simulink model "FxLMS_Sys"  (R2024b)
settings: Solver=FixedStepDiscrete  StartTime=0.0  StopTime=10  FixedStep=1/48000  RelTol=1e-3
values from neighbouring files (symbols this model uses):
  sim_p = conv(sim_s,sim_f)    [FxLMS_algo_sim.m]
  sim_s = [0.5 0.5 -0.3 -0.3 -0.2 -0.2]    [FxLMS_algo_sim.m]
undefined symbols (not defined in the file or in its folder): dspblkCoreblockFVToolHelper, gcbh
libraries: dspadpt3 x1, dspfdesign x1, dspsrcs4 x1
settings Model: PacingRate=10  Creator=shaar  LastModifiedBy=shaar

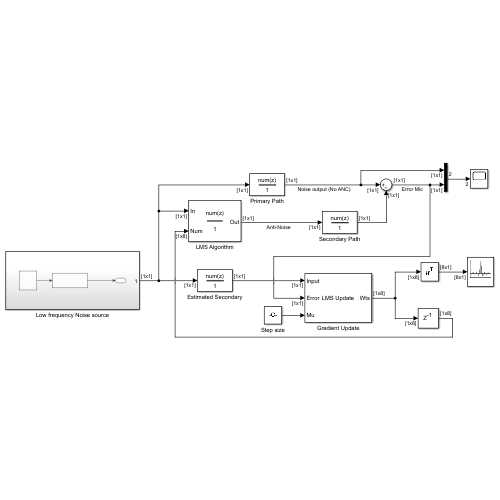
[thumbnail: Simulink's stored preview of the top-level diagram]
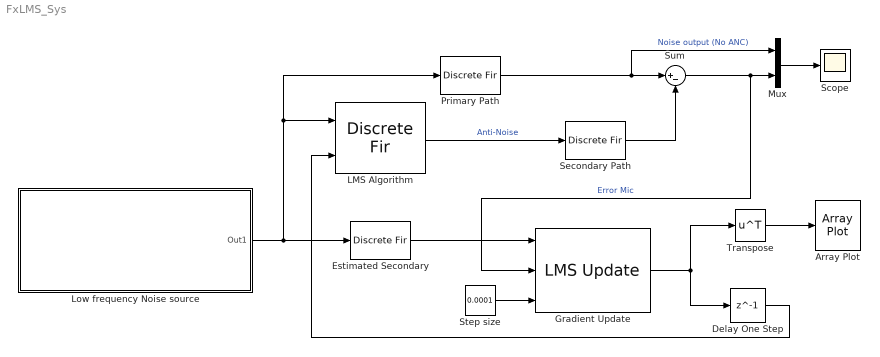
== system FxLMS_Sys ==
  Array Plot : ArrayPlot  WindowPosition=[49.000000,142.000000,800.000000,500.000000,]  ScopeFrameLocation=window  YLimits=[-0.0053 0.0054]
  Delay One Step : Delay  DelayLength=1
  Estimated Secondary : DiscreteFir  LoadFcn=dspblkCoreblockFVToolHelper(gcbh,'load');  Coefficients=sim_s
      settings: CopyFcn=dspblkCoreblockFVToolHelper(gcbh,'copy');  DeleteFcn=dspblkCoreblockFVToolHelper(gcbh,'close');  ModelCloseFcn=dspblkCoreblockFVToolHelper(gcbh,'close');  PreSaveFcn=dspblkCoreblockFVToolHelper(gcbh,'presave');  PostSaveFcn=dspblkCoreblockFVToolHelper(gcbh,'postsave');  CloseFcn=dspblkCoreblockFVToolHelper(gcbh,'close');
  Gradient Update : dspadpt3/LMS Update  Method=Normalized LMS  Length=8  NumFilters=1  StepSizeSource=Input port  StepSize=0.1  LeakageFactor=1.0  InitialConditions=0  AdaptiveFilterMode=Tapped delay-line FIR filter  EnableAdaptInput=off  EnableResetInput=off  SimulateUsing=Interpreted execution
  LMS Algorithm : DiscreteFir  LoadFcn=dspblkCoreblockFVToolHelper(gcbh,'load');  CoefSource=Input port
      settings: CopyFcn=dspblkCoreblockFVToolHelper(gcbh,'copy');  DeleteFcn=dspblkCoreblockFVToolHelper(gcbh,'close');  ModelCloseFcn=dspblkCoreblockFVToolHelper(gcbh,'close');  PreSaveFcn=dspblkCoreblockFVToolHelper(gcbh,'presave');  PostSaveFcn=dspblkCoreblockFVToolHelper(gcbh,'postsave');  CloseFcn=dspblkCoreblockFVToolHelper(gcbh,'close');  InputPortMap=u0,u1
  Low frequency Noise source : Subsystem
  Mux : Mux  Inputs=2
  Primary Path : DiscreteFir  LoadFcn=dspblkCoreblockFVToolHelper(gcbh,'load');  Coefficients=sim_p
      settings: CopyFcn=dspblkCoreblockFVToolHelper(gcbh,'copy');  DeleteFcn=dspblkCoreblockFVToolHelper(gcbh,'close');  ModelCloseFcn=dspblkCoreblockFVToolHelper(gcbh,'close');  PreSaveFcn=dspblkCoreblockFVToolHelper(gcbh,'presave');  PostSaveFcn=dspblkCoreblockFVToolHelper(gcbh,'postsave');  CloseFcn=dspblkCoreblockFVToolHelper(gcbh,'close');
  Scope : Scope
  Secondary Path : DiscreteFir  LoadFcn=dspblkCoreblockFVToolHelper(gcbh,'load');  Coefficients=sim_s
      settings: CopyFcn=dspblkCoreblockFVToolHelper(gcbh,'copy');  DeleteFcn=dspblkCoreblockFVToolHelper(gcbh,'close');  ModelCloseFcn=dspblkCoreblockFVToolHelper(gcbh,'close');  PreSaveFcn=dspblkCoreblockFVToolHelper(gcbh,'presave');  PostSaveFcn=dspblkCoreblockFVToolHelper(gcbh,'postsave');  CloseFcn=dspblkCoreblockFVToolHelper(gcbh,'close');
  Step size : Constant  Value=0.0001
  Sum : Sum  Inputs=|+-
  Transpose : Math  Operator=transpose
  wires:
  Primary Path/1 -> Mux/1, Sum/1  "Noise output (No ANC)"
  Secondary Path/1 -> Sum/2
  LMS Algorithm/1 -> Secondary Path/1  "Anti-Noise"
  Sum/1 -> Mux/2, Gradient Update/2  "Error Mic"
  Gradient Update/1 -> Delay One Step/1, Transpose/1
  Delay One Step/1 -> LMS Algorithm/2
  Transpose/1 -> Array Plot/1
  Step size/1 -> Gradient Update/3
  Estimated Secondary/1 -> Gradient Update/1
  Mux/1 -> Scope/1
  Low frequency Noise source/1(Out1) -> Estimated Secondary/1, LMS Algorithm/1, Primary Path/1

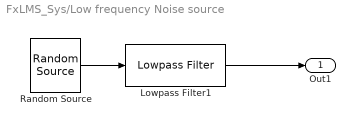
== system FxLMS_Sys/Low frequency Noise source ==
  Lowpass Filter1 : dspfdesign/Lowpass Filter  FilterType=FIR  DesignForMinimumOrder=on  FilterOrder=50  PassbandFrequency=0.0125  StopbandFrequency=0.0167  PassbandRipple=0.1  StopbandAttenuation=80  SampleRateMode=Use normalized frequency (0 to 1)  SampleRate=44100  SimulateUsing=Interpreted execution  roundingMode=Floor  coeffsDataTypeStr=fixdt(1,16)
  Random Source : dspsrcs4/Random Source  SrcType=Uniform  MinVal=-0.05  MaxVal=0.05  MeanVal=0  VarVal=1  RepMode=Specify seed  rawSeed=1  IsInherit=off  SampTime=1/48000  SampFrame=1  OutComplex=Real  DataType=double  SimulateUsing=Interpreted execution
  Out1 : Outport
  wires:
  Random Source/1 -> Lowpass Filter1/1
  Lowpass Filter1/1 -> Out1/1
